simulink model "T_outmodel"  (R2020a)
settings: Solver=VariableStepAuto  StartTime=0.0  StopTime=10.0  RelTol=1e-3
undefined symbols (not defined in the file): mc, Wc
settings Model: Creator=marce  LastModifiedBy=tkdmc

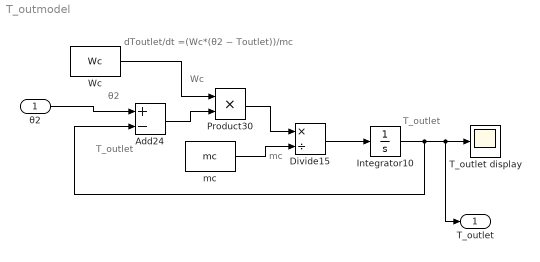
== system T_outmodel ==
  note: mc
  note: T_outlet
  note: Wc
  note: θ2
  note: T_outlet
  note: dToutlet/dt =(Wc*(θ2 − Toutlet))/mc
  θ2 : Inport
  Add24 : Sum  Inputs=+-
  Divide15 : Product  Inputs=*/
  Integrator10 : Integrator
  Product30 : Product
  T_outlet display : Scope
  Wc : Constant  Value=Wc
  mc : Constant  Value=mc
  T_outlet : Outport
  wires:
  Divide15/1 -> Integrator10/1
  Integrator10/1 -> Add24/2, T_outlet/1, T_outlet display/1
  Add24/1 -> Product30/2
  Product30/1 -> Divide15/1
  θ2/1 -> Add24/1
  Wc/1 -> Product30/1
  mc/1 -> Divide15/2
